simulink library "LIB_FDI"  (Simulink 8.8)
settings: Solver=VariableStepAuto  StartTime=0.0  StopTime=10.0  RelTol=1e-3
settings Model: Creator=alger  LastModifiedBy=alger

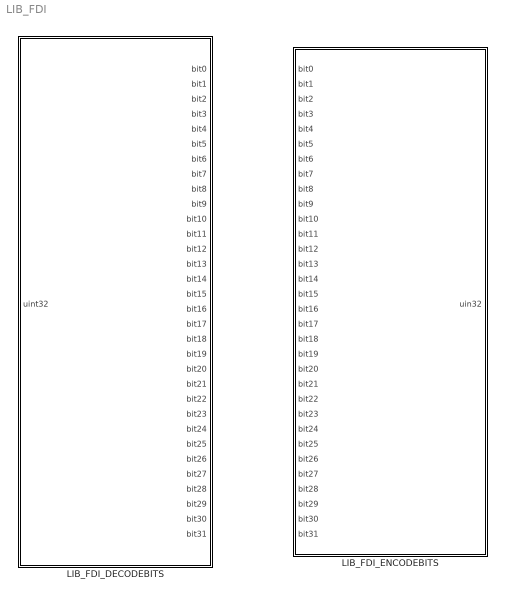
== system LIB_FDI ==
  LIB_FDI_DECODEBITS : Subsystem  mask(decodes a uint32 value into individual bits){}
      mask help: A library block to perform bit level decoding
  LIB_FDI_ENCODEBITS : Subsystem  mask(Encodes individual bits into uint32){}
      mask help: A library block to perform bit level encoding

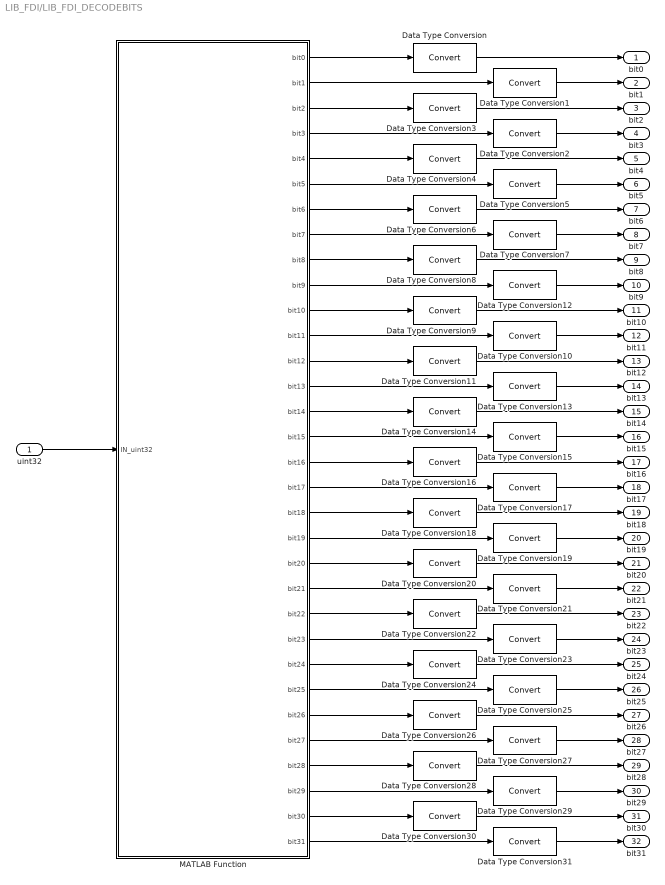
== system LIB_FDI/LIB_FDI_DECODEBITS ==
  uint32 : Inport  OutDataTypeStr=uint32
  Data Type Conversion{,1..31} (32 alike) : DataTypeConversion
  MATLAB Function : MATLAB Function  TreatAsAtomicUnit=on
  bit0 : Outport  OutDataTypeStr=boolean
  bit1 : Outport  Port=2  OutDataTypeStr=boolean
  bit2 : Outport  Port=3  OutDataTypeStr=boolean
  bit3 : Outport  Port=4  OutDataTypeStr=boolean
  bit4 : Outport  Port=5  OutDataTypeStr=boolean
  bit5 : Outport  Port=6  OutDataTypeStr=boolean
  bit6 : Outport  Port=7  OutDataTypeStr=boolean
  bit7 : Outport  Port=8  OutDataTypeStr=boolean
  bit8 : Outport  Port=9  OutDataTypeStr=boolean
  bit9 : Outport  Port=10  OutDataTypeStr=boolean
  bit10 : Outport  Port=11  OutDataTypeStr=boolean
  bit11 : Outport  Port=12  OutDataTypeStr=boolean
  bit12 : Outport  Port=13  OutDataTypeStr=boolean
  bit13 : Outport  Port=14  OutDataTypeStr=boolean
  bit14 : Outport  Port=15  OutDataTypeStr=boolean
  bit15 : Outport  Port=16  OutDataTypeStr=boolean
  bit16 : Outport  Port=17  OutDataTypeStr=boolean
  bit17 : Outport  Port=18  OutDataTypeStr=boolean
  bit18 : Outport  Port=19  OutDataTypeStr=boolean
  bit19 : Outport  Port=20  OutDataTypeStr=boolean
  bit20 : Outport  Port=21  OutDataTypeStr=boolean
  bit21 : Outport  Port=22  OutDataTypeStr=boolean
  bit22 : Outport  Port=23  OutDataTypeStr=boolean
  bit23 : Outport  Port=24  OutDataTypeStr=boolean
  bit24 : Outport  Port=25  OutDataTypeStr=boolean
  bit25 : Outport  Port=26  OutDataTypeStr=boolean
  bit26 : Outport  Port=27  OutDataTypeStr=boolean
  bit27 : Outport  Port=28  OutDataTypeStr=boolean
  bit28 : Outport  Port=29  OutDataTypeStr=boolean
  bit29 : Outport  Port=30  OutDataTypeStr=boolean
  bit30 : Outport  Port=31  OutDataTypeStr=boolean
  bit31 : Outport  Port=32  OutDataTypeStr=boolean
  wires:
  MATLAB Function/28(bit27) -> Data Type Conversion27/1
  MATLAB Function/30(bit29) -> Data Type Conversion29/1
  MATLAB Function/24(bit23) -> Data Type Conversion23/1
  MATLAB Function/22(bit21) -> Data Type Conversion21/1
  MATLAB Function/32(bit31) -> Data Type Conversion31/1
  MATLAB Function/8(bit7) -> Data Type Conversion7/1
  MATLAB Function/14(bit13) -> Data Type Conversion13/1
  MATLAB Function/6(bit5) -> Data Type Conversion5/1
  MATLAB Function/16(bit15) -> Data Type Conversion15/1
  MATLAB Function/12(bit11) -> Data Type Conversion10/1
  MATLAB Function/10(bit9) -> Data Type Conversion12/1
  MATLAB Function/20(bit19) -> Data Type Conversion19/1
  MATLAB Function/18(bit17) -> Data Type Conversion17/1
  MATLAB Function/26(bit25) -> Data Type Conversion25/1
  MATLAB Function/31(bit30) -> Data Type Conversion30/1
  MATLAB Function/29(bit28) -> Data Type Conversion28/1
  MATLAB Function/27(bit26) -> Data Type Conversion26/1
  MATLAB Function/25(bit24) -> Data Type Conversion24/1
  MATLAB Function/23(bit22) -> Data Type Conversion22/1
  MATLAB Function/21(bit20) -> Data Type Conversion20/1
  MATLAB Function/19(bit18) -> Data Type Conversion18/1
  MATLAB Function/17(bit16) -> Data Type Conversion16/1
  MATLAB Function/15(bit14) -> Data Type Conversion14/1
  MATLAB Function/13(bit12) -> Data Type Conversion11/1
  MATLAB Function/11(bit10) -> Data Type Conversion9/1
  MATLAB Function/9(bit8) -> Data Type Conversion8/1
  MATLAB Function/7(bit6) -> Data Type Conversion6/1
  MATLAB Function/5(bit4) -> Data Type Conversion4/1
  MATLAB Function/3(bit2) -> Data Type Conversion3/1
  MATLAB Function/1(bit0) -> Data Type Conversion/1
  MATLAB Function/4(bit3) -> Data Type Conversion2/1
  MATLAB Function/2(bit1) -> Data Type Conversion1/1
  uint32/1 -> MATLAB Function/1(IN_uint32)
  Data Type Conversion/1 -> bit0/1
  Data Type Conversion1/1 -> bit1/1
  Data Type Conversion2/1 -> bit3/1
  Data Type Conversion3/1 -> bit2/1
  Data Type Conversion4/1 -> bit4/1
  Data Type Conversion5/1 -> bit5/1
  Data Type Conversion6/1 -> bit6/1
  Data Type Conversion7/1 -> bit7/1
  Data Type Conversion8/1 -> bit8/1
  Data Type Conversion9/1 -> bit10/1
  Data Type Conversion10/1 -> bit11/1
  Data Type Conversion11/1 -> bit12/1
  Data Type Conversion12/1 -> bit9/1
  Data Type Conversion13/1 -> bit13/1
  Data Type Conversion14/1 -> bit14/1
  Data Type Conversion15/1 -> bit15/1
  Data Type Conversion16/1 -> bit16/1
  Data Type Conversion17/1 -> bit17/1
  Data Type Conversion18/1 -> bit18/1
  Data Type Conversion19/1 -> bit19/1
  Data Type Conversion20/1 -> bit20/1
  Data Type Conversion21/1 -> bit21/1
  Data Type Conversion22/1 -> bit22/1
  Data Type Conversion23/1 -> bit23/1
  Data Type Conversion24/1 -> bit24/1
  Data Type Conversion25/1 -> bit25/1
  Data Type Conversion26/1 -> bit26/1
  Data Type Conversion27/1 -> bit27/1
  Data Type Conversion28/1 -> bit28/1
  Data Type Conversion29/1 -> bit29/1
  Data Type Conversion30/1 -> bit30/1
  Data Type Conversion31/1 -> bit31/1

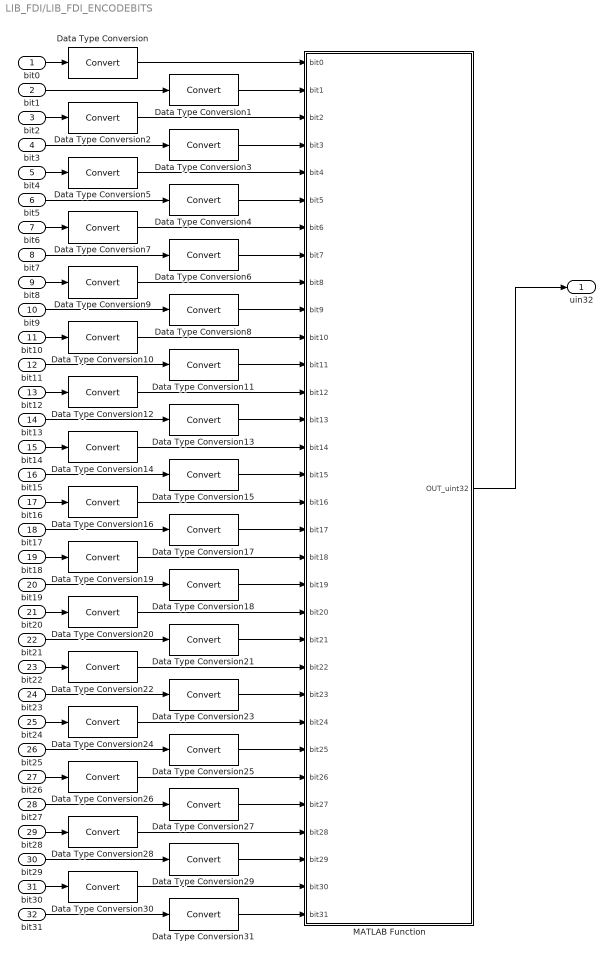
== system LIB_FDI/LIB_FDI_ENCODEBITS ==
  bit0 : Inport  OutDataTypeStr=boolean
  bit1 : Inport  Port=2  OutDataTypeStr=boolean
  bit2 : Inport  Port=3  OutDataTypeStr=boolean
  bit3 : Inport  Port=4  OutDataTypeStr=boolean
  bit4 : Inport  Port=5  OutDataTypeStr=boolean
  bit5 : Inport  Port=6  OutDataTypeStr=boolean
  bit6 : Inport  Port=7  OutDataTypeStr=boolean
  bit7 : Inport  Port=8  OutDataTypeStr=boolean
  bit8 : Inport  Port=9  OutDataTypeStr=boolean
  bit9 : Inport  Port=10  OutDataTypeStr=boolean
  bit10 : Inport  Port=11  OutDataTypeStr=boolean
  bit11 : Inport  Port=12  OutDataTypeStr=boolean
  bit12 : Inport  Port=13  OutDataTypeStr=boolean
  bit13 : Inport  Port=14  OutDataTypeStr=boolean
  bit14 : Inport  Port=15  OutDataTypeStr=boolean
  bit15 : Inport  Port=16  OutDataTypeStr=boolean
  bit16 : Inport  Port=17  OutDataTypeStr=boolean
  bit17 : Inport  Port=18  OutDataTypeStr=boolean
  bit18 : Inport  Port=19  OutDataTypeStr=boolean
  bit19 : Inport  Port=20  OutDataTypeStr=boolean
  bit20 : Inport  Port=21  OutDataTypeStr=boolean
  bit21 : Inport  Port=22  OutDataTypeStr=boolean
  bit22 : Inport  Port=23  OutDataTypeStr=boolean
  bit23 : Inport  Port=24  OutDataTypeStr=boolean
  bit24 : Inport  Port=25  OutDataTypeStr=boolean
  bit25 : Inport  Port=26  OutDataTypeStr=boolean
  bit26 : Inport  Port=27  OutDataTypeStr=boolean
  bit27 : Inport  Port=28  OutDataTypeStr=boolean
  bit28 : Inport  Port=29  OutDataTypeStr=boolean
  bit29 : Inport  Port=30  OutDataTypeStr=boolean
  bit30 : Inport  Port=31  OutDataTypeStr=boolean
  bit31 : Inport  Port=32  OutDataTypeStr=boolean
  Data Type Conversion{,1..31} (32 alike) : DataTypeConversion
  MATLAB Function : MATLAB Function  TreatAsAtomicUnit=on
  uin32 : Outport  OutDataTypeStr=uint32
  wires:
  bit4/1 -> Data Type Conversion5/1
  bit16/1 -> Data Type Conversion16/1
  bit2/1 -> Data Type Conversion2/1
  bit6/1 -> Data Type Conversion7/1
  bit22/1 -> Data Type Conversion22/1
  bit9/1 -> Data Type Conversion8/1
  bit5/1 -> Data Type Conversion4/1
  bit1/1 -> Data Type Conversion1/1
  bit3/1 -> Data Type Conversion3/1
  bit12/1 -> Data Type Conversion12/1
  bit10/1 -> Data Type Conversion10/1
  bit14/1 -> Data Type Conversion14/1
  bit26/1 -> Data Type Conversion26/1
  bit18/1 -> Data Type Conversion19/1
  bit24/1 -> Data Type Conversion24/1
  bit28/1 -> Data Type Conversion28/1
  bit20/1 -> Data Type Conversion20/1
  bit30/1 -> Data Type Conversion30/1
  MATLAB Function/1(OUT_uint32) -> uin32/1
  bit11/1 -> Data Type Conversion11/1
  bit13/1 -> Data Type Conversion13/1
  bit15/1 -> Data Type Conversion15/1
  bit23/1 -> Data Type Conversion23/1
  bit21/1 -> Data Type Conversion21/1
  bit25/1 -> Data Type Conversion25/1
  bit17/1 -> Data Type Conversion17/1
  bit7/1 -> Data Type Conversion6/1
  bit27/1 -> Data Type Conversion27/1
  bit29/1 -> Data Type Conversion29/1
  bit19/1 -> Data Type Conversion18/1
  bit31/1 -> Data Type Conversion31/1
  bit8/1 -> Data Type Conversion9/1
  bit0/1 -> Data Type Conversion/1
  Data Type Conversion/1 -> MATLAB Function/1(bit0)
  Data Type Conversion1/1 -> MATLAB Function/2(bit1)
  Data Type Conversion2/1 -> MATLAB Function/3(bit2)
  Data Type Conversion3/1 -> MATLAB Function/4(bit3)
  Data Type Conversion4/1 -> MATLAB Function/6(bit5)
  Data Type Conversion5/1 -> MATLAB Function/5(bit4)
  Data Type Conversion6/1 -> MATLAB Function/8(bit7)
  Data Type Conversion7/1 -> MATLAB Function/7(bit6)
  Data Type Conversion8/1 -> MATLAB Function/10(bit9)
  Data Type Conversion9/1 -> MATLAB Function/9(bit8)
  Data Type Conversion10/1 -> MATLAB Function/11(bit10)
  Data Type Conversion11/1 -> MATLAB Function/12(bit11)
  Data Type Conversion12/1 -> MATLAB Function/13(bit12)
  Data Type Conversion13/1 -> MATLAB Function/14(bit13)
  Data Type Conversion14/1 -> MATLAB Function/15(bit14)
  Data Type Conversion15/1 -> MATLAB Function/16(bit15)
  Data Type Conversion16/1 -> MATLAB Function/17(bit16)
  Data Type Conversion17/1 -> MATLAB Function/18(bit17)
  Data Type Conversion18/1 -> MATLAB Function/20(bit19)
  Data Type Conversion19/1 -> MATLAB Function/19(bit18)
  Data Type Conversion20/1 -> MATLAB Function/21(bit20)
  Data Type Conversion21/1 -> MATLAB Function/22(bit21)
  Data Type Conversion22/1 -> MATLAB Function/23(bit22)
  Data Type Conversion23/1 -> MATLAB Function/24(bit23)
  Data Type Conversion24/1 -> MATLAB Function/25(bit24)
  Data Type Conversion25/1 -> MATLAB Function/26(bit25)
  Data Type Conversion26/1 -> MATLAB Function/27(bit26)
  Data Type Conversion27/1 -> MATLAB Function/28(bit27)
  Data Type Conversion28/1 -> MATLAB Function/29(bit28)
  Data Type Conversion29/1 -> MATLAB Function/30(bit29)
  Data Type Conversion30/1 -> MATLAB Function/31(bit30)
  Data Type Conversion31/1 -> MATLAB Function/32(bit31)

== matlab function LIB_FDI_DECODEBITS/MATLAB Function ==
  data: IN_uint32 input double; bit0 output double; bit1 output double; bit2 output double; bit3 output double; bit4 output double; bit5 output double; bit6 output double; bit7 output double; bit8 output double; bit9 output double; bit10 output double; bit11 output double; bit12 output double; bit13 output double; bit14 output double; bit15 output double; bit16 output double; bit17 output double; bit18 output double; bit19 output double; bit20 output double; bit21 output double; bit22 output double; bit23 output double; bit24 output double; bit25 output double; bit26 output double; bit27 output double; bit28 output double; bit29 output double; bit30 output double; bit31 output double
function [ bit0 , ...
    bit1 , ...
    bit2 , ...
    bit3 , ...
    bit4 , ...
    bit5 , ...
    bit6 , ...
    bit7 , ...
    bit8 , ...
    bit9 , ...
    bit10, ...
    bit11, ...
    bit12, ...
    bit13, ...
    bit14, ...
    bit15, ...
    bit16, ...
    bit17, ...
    bit18, ...
    bit19, ...
    bit20, ...
    bit21, ...
    bit22, ...
    bit23, ...
    bit24, ...
    bit25, ...
    bit26, ...
    bit27, ...
    bit28, ...
    bit29, ...
    bit30, ...
    bit31 ] = call_decodebits( IN_uint32 )
  
  
  [ bit0 , ...
    bit1 , ...
    bit2 , ...
    bit3 , ...
    bit4 , ...
    bit5 , ...
    bit6 , ...
    bit7 , ...
    bit8 , ...
    bit9 , ...
    bit10, ...
    bit11, ...
    bit12, ...
    bit13, ...
    bit14, ...
    bit15, ...
    bit16, ...
    bit17, ...
    bit18, ...
    bit19, ...
    bit20, ...
    bit21, ...
    bit22, ...
    bit23, ...
    bit24, ...
    bit25, ...
    bit26, ...
    bit27, ...
    bit28, ...
    bit29, ...
    bit30, ...
    bit31 ] = decodebits( IN_uint32 );
end

== matlab function LIB_FDI_ENCODEBITS/MATLAB Function ==
  data: bit0 input uint32; OUT_uint32 output uint32; bit1 input boolean; bit2 input boolean; bit3 input boolean; bit4 input boolean; bit5 input boolean; bit6 input boolean; bit7 input boolean; bit8 input boolean; bit9 input boolean; bit10 input boolean; bit11 input boolean; bit12 input boolean; bit13 input boolean; bit14 input boolean; bit15 input boolean; bit16 input boolean; bit17 input boolean; bit18 input boolean; bit19 input boolean; bit20 input boolean; bit21 input boolean; bit22 input boolean; bit23 input boolean; bit24 input boolean; bit25 input boolean; bit26 input boolean; bit27 input boolean; bit28 input boolean; bit29 input boolean; bit30 input boolean; bit31 input boolean
function OUT_uint32  = call_encodebits(bit0 , ...
                                   bit1 , ...
                                   bit2 , ...
                                   bit3 , ...
                                   bit4 , ...
                                   bit5 , ...
                                   bit6 , ...
                                   bit7 , ...
                                   bit8 , ...
                                   bit9 , ...
                                   bit10, ...
                                   bit11, ...
                                   bit12, ...
                                   bit13, ...
                                   bit14, ...
                                   bit15, ...
                                   bit16, ...
                                   bit17, ...
                                   bit18, ...
                                   bit19, ...
                                   bit20, ...
                                   bit21, ...
                                   bit22, ...
                                   bit23, ...
                                   bit24, ...
                                   bit25, ...
                                   bit26, ...
                                   bit27, ...
                                   bit28, ...
                                   bit29, ...
                                   bit30, ...
                                   bit31)
                                 
%#codegen                                 
[OUT_uint32] = encodebits(bit0 , ...
                                   bit1 , ...
                                   bit2 , ...
                                   bit3 , ...
                                   bit4 , ...
                                   bit5 , ...
                                   bit6 , ...
                                   bit7 , ...
                                   bit8 , ...
                                   bit9 , ...
                                   bit10, ...
                                   bit11, ...
                                   bit12, ...
                                   bit13, ...
                                   bit14, ...
                                   bit15, ...
                                   bit16, ...
                                   bit17, ...
                                   bit18, ...
                                   bit19, ...
                                   bit20, ...
                                   bit21, ...
                                   bit22, ...
                                   bit23, ...
                                   bit24, ...
                                   bit25, ...
                                   bit26, ...
                                   bit27, ...
                                   bit28, ...
                                   bit29, ...
                                   bit30, ...
                                   bit31);
end
